simulink model "visual_sim"  (R2020a)
settings: Solver=ode3  StartTime=0.0  StopTime=Inf  RelTol=1e-3  EnableMultiTasking=on
undefined symbols (not defined in the file or in its folder): Rec, SDTV
libraries: dspsigops x6, simulink x3, visionstatistics x1, visionanalysis x1, visionconversions x1, embdlinuxlib x1
settings Model: FPTRunName=Active  ExtModeTrigDuration=2  Creator=ianli  LastModifiedBy=vyvo9
settings SolverCC: PositivePriorityOrder=on
settings DataIOCC: LimitDataPoints=on  SaveFormat=Array
settings OptimizationCC: ExpressionDepthLimit=2147483647  LifeSpan=Inf  MaxStackSize=64
settings DebuggingCC: UnderspecifiedInitializationDetection=Classic  MergeDetectMultiDrivingBlocksExec=none  FcnCallInpInsideContextMsg=warning  AllowSymbolicDim=off  StateNameClashWarn=warning  SFUnexpectedBacktrackingDiag=warning  SFNoUnconditionalDefaultTransitionDiag=warning  SFExecutionAtInitializationDiag=none  ArithmeticOperatorsInVariantConditions=warning
settings HardwareCC: ProdBitPerPointer=32  ProdBitPerSizeT=32  ProdBitPerPtrDiffT=32  ProdLargestAtomicInteger=Long  ProdLargestAtomicFloat=Double  ProdWordSize=32  ProdHWDeviceType=ARM Compatible->ARM Cortex  UseEmbeddedCoderFeatures=off
settings ModelReferenceCC: PropagateSignalLabelsOutOfModel=off
settings SFSimCC: SimUseLocalCustomCode=off  CustomCodeUndefinedFunction=UseInterfaceOnly
settings RTWCC: SystemTargetFile=ert.tlc  HardwareBoard=Raspberry Pi  TemplateMakefile=ert_default_tmf  GenerateReport=on  RTWVerbose=off  RTWUseLocalCustomCode=off  Toolchain=GNU GCC Raspberry Pi  BuildConfiguration=Faster Runs  LaunchReport=on
settings CodeAppCC: ForceParamTrailComments=on  OperatorAnnotations=on  StateflowObjectComments=on  MATLABSourceComments=on
settings ERTTargetCC: MultiwordLength=2048  ERTCustomFileBanners=off  SupportContinuousTime=on  SupportNonInlinedSFcns=on  RemoveResetFunc=off  SupportVariableSizeSignals=on  ModelStepFunctionPrototypeControlCompliant=off
settings ConfigComp: CovMetricSettings=dw  CovHtmlReporting=on  CovSaveCumulativeToWorkspaceVar=on  CovSaveSingleToWorkspaceVar=on  CovExternalEMLEnable=off  CovSFcnEnable=off

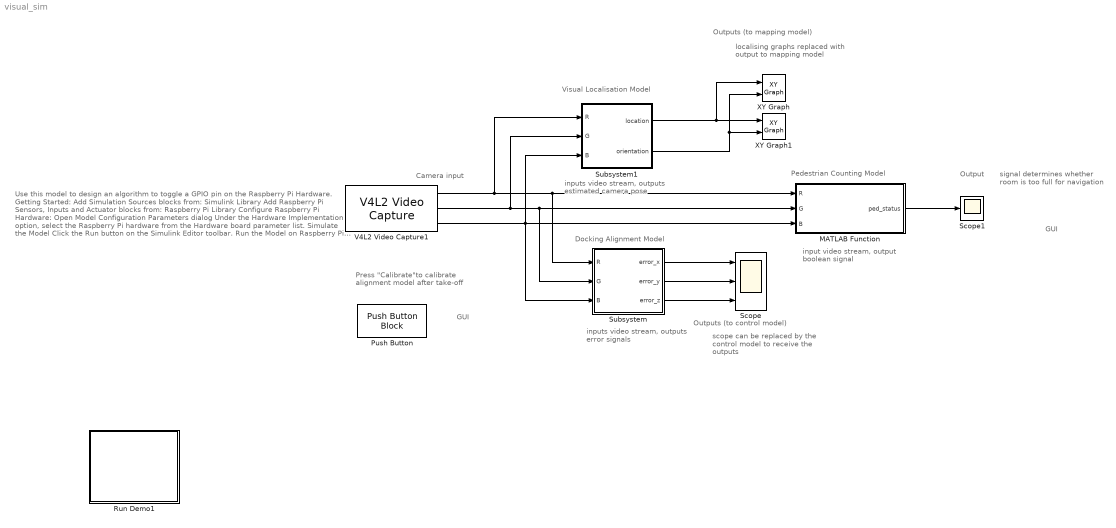
== system visual_sim ==
  note: Outputs (to control model)
  note: inputs video stream,
      | outputs error signals
  note: Camera input
  note: Docking Alignment Model
  note: Press "Calibrate"to calibrate alignment model after take-off
  note: scope can be replaced by the control model to receive the outputs
  note: GUI
  note: input video stream,
      | output boolean signal
  note: Use this model to design an algorithm to toggle a GPIO pin on the Raspberry Pi Hardware.
      |
      | Getting Started:
      |
      | Add Simulation Sources blocks from:
      | Simulink Library
      | Add Raspberry Pi Sensors, Inputs and Actuator blocks from:
      | Raspberry Pi Library
      |
      | Configure Raspberry Pi Hardware:
      |
      | Open Model Configuration Parameters dialog
      | Under the Hardware Implementation option, select the Raspberry Pi hardware from the Hardware board parameter list.
      |
      | Simulate the Model
      |
      | Click the Run button on the Simulink Editor toolbar.
      |
      | Run the Model on Raspberry Pi Hardware
      |
      | In the Hardware tab, click Build, Deploy & Start
      |
      | Other Things to Try:
      |
      | Create and run a model that repeatedly brightens and dims an LED. Hint: Use PWM block as an Raspberry Pi actuator.
  note: Visual Localisation Model
  note: inputs video stream,
      | outputs estimated camera pose
  note: Output
  note: signal determines whether room is too full for navigation
  note: Pedestrian Counting Model
  note: Outputs (to mapping model)
  note: localising graphs replaced with output to mapping model
  note: GUI
  MATLAB Function : MATLAB Function  TreatAsAtomicUnit=on
  Push Button : PushButtonBlock  ButtonText=Callibrate
  Run Demo1 : Subsystem  Description=Controls host-side RTDX processing.
      mask Display: pic=imread('raspberrypiBuildDeployAndStart.png');image(pic);
  Scope : Scope  NumInputPorts=3
  Scope1 : Scope
  Subsystem : Subsystem
  Subsystem1 : Subsystem
  V4L2 Video Capture1 : embdlinuxlib/V4L2 Video Capture  m_devName='/dev/video0'  roi=[0, 0, 640, 480]  imSizeSelection=640x480  imSize=[640, 480]  pixelFormat=RGB  pixelOrder=Planar  sampleTime=1/10  simOutput=Colorbars  blockPlatform=Raspberry Pi
      settings: SourceProductBaseCode=SC_BEAGLEBONE_BLUE,RASPPI
  XY Graph : simulink/Sinks/XY Graph  xmin=-1  xmax=1  ymin=-1  ymax=1  st=-1
  XY Graph1 : simulink/Sinks/XY Graph  xmin=-1  xmax=1  ymin=-1  ymax=1  st=-1
  wires:
  Subsystem/1(error_x) -> Scope/1
  Subsystem/2(error_y) -> Scope/2
  Subsystem/3(error_z) -> Scope/3
  V4L2 Video Capture1/2 -> Subsystem1/2(G), Subsystem/2(G), MATLAB Function/2(G)
  V4L2 Video Capture1/3 -> MATLAB Function/3(B), Subsystem/3(B), Subsystem1/3(B)
  V4L2 Video Capture1/1 -> Subsystem1/1(R), Subsystem/1(R), MATLAB Function/1(R)
  MATLAB Function/1(ped_status) -> Scope1/1
  Subsystem1/1(location) -> XY Graph1/1, XY Graph/1
  Subsystem1/2(orientation) -> XY Graph1/2, XY Graph/2

== system visual_sim/Run Demo1 ==

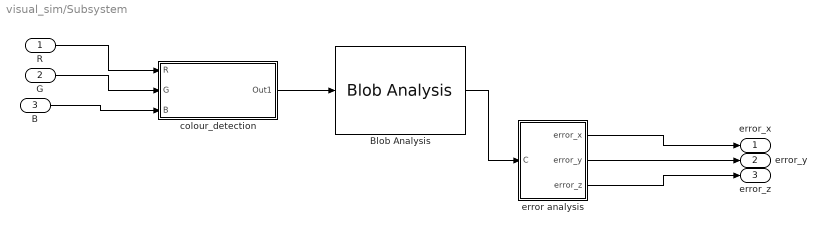
== system visual_sim/Subsystem ==
  R : Inport
  G : Inport  Port=2
  B : Inport  Port=3
  Blob Analysis : visionstatistics/Blob Analysis  Tag=vipblks_row_conv  area=off  centroid=on  bBox=off  majorAxis=off  minorAxis=off  angle=off  eccentricity=off  equivDiameterSq=off  extent=off  perimeter=off  outDT=double  conn=8  isLabel=off  maxBlobs=3  warnIfNumBlobsExceeded=on  isCount=off  useMinArea=off  minArea=0  useMaxArea=off  maxArea=intmax('uint32')  excludeBorderBlob=off  isOutVarDim=off  isFill=on  fillValues=-1  roundingMode=Floor  overflowMode=off  prodOutputMode=Binary point scaling  prodOutputWordLength=32  prodOutputFracLength=16  accumMode=Binary point scaling  accumWordLength=32  accumFracLength=0  outputMode=Binary point scaling  outputWordLength=32  outputFracLength=16  firstCoeffMode=Binary point scaling  firstCoeffWordLength=16  firstCoeffFracLength=14  secondCoeffMode=Binary point scaling  secondCoeffWordLength=32  secondCoeffFracLength=16
  colour_detection : Subsystem
  error analysis : Subsystem
  error_x : Outport
  error_y : Outport  Port=2
  error_z : Outport  Port=3
  wires:
  Blob Analysis/1 -> error analysis/1(C)
  colour_detection/1(Out1) -> Blob Analysis/1
  error analysis/1(error_x) -> error_x/1
  error analysis/2(error_y) -> error_y/1
  error analysis/3(error_z) -> error_z/1
  R/1 -> colour_detection/1(R)
  G/1 -> colour_detection/2(G)
  B/1 -> colour_detection/3(B)

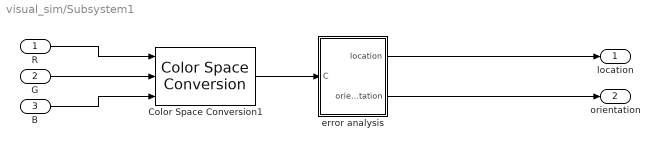
== system visual_sim/Subsystem1 ==
  R : Inport
  G : Inport  Port=2
  B : Inport  Port=3
  Color Space Conversion1 : visionconversions/Color Space  Conversion  conversion=Obsolete  conversionActive=R'G'B' to intensity  wp_str=D65  rec=Rec. 601 (SDTV)  sys=1125/60/2:1  imagePorts=Separate color signals
  error analysis : Subsystem
  location : Outport
  orientation : Outport  Port=2
  wires:
  error analysis/1(location) -> location/1
  error analysis/2(orientation) -> orientation/1
  R/1 -> Color Space Conversion1/1
  G/1 -> Color Space Conversion1/2
  B/1 -> Color Space Conversion1/3
  Color Space Conversion1/1 -> error analysis/1(C)

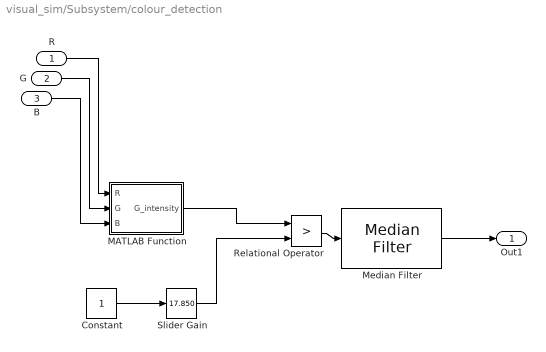
== system visual_sim/Subsystem/colour_detection ==
  R : Inport
  G : Inport  Port=2
  B : Inport  Port=3
  Constant : Constant
  MATLAB Function : MATLAB Function  TreatAsAtomicUnit=on
  Median Filter : visionanalysis/Median Filter  nghbood=[3 3]  outSize=Same as input port I  padType=Constant  padSrc=Specify via dialog  padVal=0  roundingMode=Floor  overflowMode=off
      settings: SourceProductBaseCode=VP
  Relational Operator : RelationalOperator  Operator=>  OutDataTypeStr=boolean  RndMeth=Simplest
  Slider Gain : simulink/Math Operations/Slider Gain  gain=17.850  low=0  high=255
  Out1 : Outport
  wires:
  Slider Gain/1 -> Relational Operator/2
  Constant/1 -> Slider Gain/1
  MATLAB Function/1(G_intensity) -> Relational Operator/1
  G/1 -> MATLAB Function/2(G)
  B/1 -> MATLAB Function/3(B)
  Median Filter/1 -> Out1/1
  R/1 -> MATLAB Function/1(R)
  Relational Operator/1 -> Median Filter/1

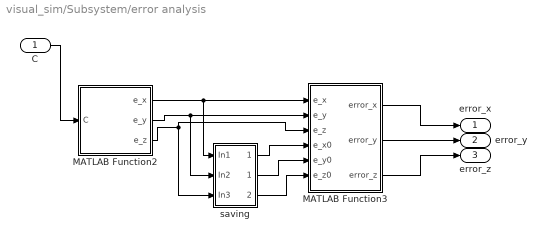
== system visual_sim/Subsystem/error analysis ==
  C : Inport
  MATLAB Function2 : MATLAB Function  TreatAsAtomicUnit=on
  MATLAB Function3 : MATLAB Function  TreatAsAtomicUnit=on
  saving : Subsystem
  error_x : Outport
  error_y : Outport  Port=2
  error_z : Outport  Port=3
  wires:
  MATLAB Function2/2(e_y) -> MATLAB Function3/2(e_y), saving/2(In2)
  MATLAB Function2/1(e_x) -> saving/1(In1), MATLAB Function3/1(e_x)
  saving/3(" 2") -> MATLAB Function3/6(e_z0)
  saving/2(" 1") -> MATLAB Function3/5(e_y0)
  MATLAB Function2/3(e_z) -> MATLAB Function3/3(e_z), saving/3(In3)
  saving/1(" ") -> MATLAB Function3/4(e_x0)
  MATLAB Function3/1(error_x) -> error_x/1
  MATLAB Function3/3(error_z) -> error_z/1
  MATLAB Function3/2(error_y) -> error_y/1
  C/1 -> MATLAB Function2/1(C)

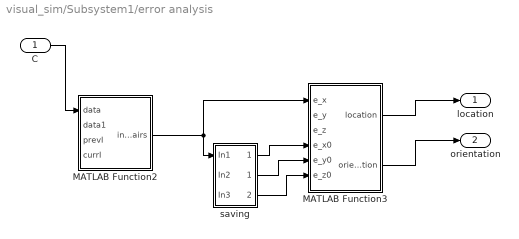
== system visual_sim/Subsystem1/error analysis ==
  C : Inport
  MATLAB Function2 : MATLAB Function  TreatAsAtomicUnit=on
  MATLAB Function3 : MATLAB Function  TreatAsAtomicUnit=on
  saving : Subsystem
  location : Outport
  orientation : Outport  Port=2
  wires:
  ? -> MATLAB Function3/2(e_y), saving/2(In2)
  MATLAB Function2/1(indexPairs) -> MATLAB Function3/1(e_x), saving/1(In1)
  saving/3(" 2") -> MATLAB Function3/6(e_z0)
  saving/2(" 1") -> MATLAB Function3/5(e_y0)
  ? -> MATLAB Function3/3(e_z), saving/3(In3)
  saving/1(" ") -> MATLAB Function3/4(e_x0)
  MATLAB Function3/1(location) -> location/1
  MATLAB Function3/2(orientation) -> orientation/1
  C/1 -> MATLAB Function2/1(data)

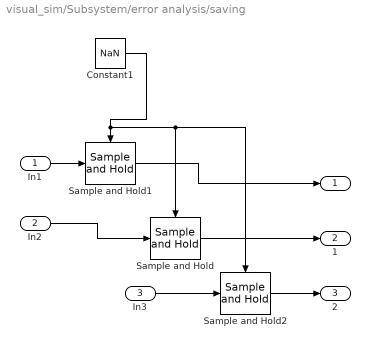
== system visual_sim/Subsystem/error analysis/saving ==
  In1 : Inport
  In2 : Inport  Port=2
  In3 : Inport  Port=3
  Constant1 : Constant  Value=NaN
  Sample and Hold : dspsigops/Sample and Hold  trig=Rising edge  initCond=0  latchinput=off
  Sample and Hold1 : dspsigops/Sample and Hold  trig=Rising edge  initCond=0  latchinput=off
  Sample and Hold2 : dspsigops/Sample and Hold  trig=Rising edge  initCond=0  latchinput=off
  " " : Outport
  " 1" : Outport  Port=2
  " 2" : Outport  Port=3
  wires:
  Sample and Hold1/1 -> " "/1
  In1/1 -> Sample and Hold1/1
  In2/1 -> Sample and Hold/1
  Sample and Hold/1 -> " 1"/1
  Sample and Hold2/1 -> " 2"/1
  In3/1 -> Sample and Hold2/1
  Constant1/1 -> Sample and Hold2/Trigger, Sample and Hold/Trigger, Sample and Hold1/Trigger

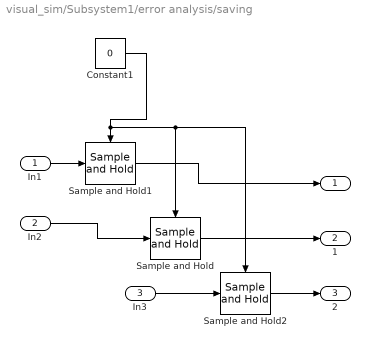
== system visual_sim/Subsystem1/error analysis/saving ==
  In1 : Inport
  In2 : Inport  Port=2
  In3 : Inport  Port=3
  Constant1 : Constant  Value=0
  Sample and Hold : dspsigops/Sample and Hold  trig=Rising edge  initCond=0  latchinput=off
  Sample and Hold1 : dspsigops/Sample and Hold  trig=Rising edge  initCond=0  latchinput=off
  Sample and Hold2 : dspsigops/Sample and Hold  trig=Rising edge  initCond=0  latchinput=off
  " " : Outport
  " 1" : Outport  Port=2
  " 2" : Outport  Port=3
  wires:
  Sample and Hold1/1 -> " "/1
  In1/1 -> Sample and Hold1/1
  In2/1 -> Sample and Hold/1
  Sample and Hold/1 -> " 1"/1
  Sample and Hold2/1 -> " 2"/1
  In3/1 -> Sample and Hold2/1
  Constant1/1 -> Sample and Hold2/Trigger, Sample and Hold/Trigger, Sample and Hold1/Trigger

== matlab function visual_sim/Subsystem/colour_detection/MATLAB Function ==
  data: R input; G_intensity output; G input; B input
function G_intensity  = fcn(R,G,B)

G_intensity = G - R./2 - B./2;

== matlab function visual_sim/Subsystem/error analysis/MATLAB Function2 ==
  data: C input; e_x output; e_y output; e_z output
function [e_x, e_y, e_z] = distances(C) % note everything is in pixels

% input C gives a 3-by-2 matrix in in the form [x1 y1 ; x2 y2 ; x3 y3] of
% the coordinates of the centroids
% (possible input that can be obtained from blob analysis is also blob area
% which can be used to identify the different blobs)
if length(C)==3
    C_sorted = sortrows(C); % sort so rows 1-3 correspond to blobs from L-R
    % NB blob 1,3 are the back markers, blob 3 is the front marker
    e_x = (C_sorted(3,1)+C_sorted(2,1))/2-C_sorted(2,1); %+ve error - too far right
    e_z = (C_sorted(3,2)+C_sorted(2,2))/2-C_sorted(2,2); %+ve error - too high
    e_y = (C_sorted(3,1)-C_sorted(1,1)); % relative distance between poles in pixels
end

== matlab function visual_sim/Subsystem/error analysis/MATLAB Function3 ==
  data: e_x input; e_y input; error_x output; error_y output; e_z input; e_x0 input; e_y0 input; e_z0 input; error_z output
function [error_x,error_y,error_z] = fcn(e_x,e_y,e_z,e_x0,e_y0,e_z0)

error_x = e_x-e_x0;
error_z = e_z-e_z0;
error_y = e_y-e_y0;

== matlab function visual_sim/MATLAB Function ==
  data: R input; ped_status output; G input; B input
function ped_status = PedestrianTracking(R, G, B)
[obj, tracks, full, FrameWithTracker] = PedestrianTracker();
objs = obj;
trackss = tracks;
ped_status = [full, FrameWithTracker];

== matlab function visual_sim/Subsystem1/error analysis/MATLAB Function2 ==
  data: data input; indexPairs output; data1 input; prevI input; currI input
function indexPairs  = fcn(data, data1, prevI, currI)

prevPoints = detectSURFFeatures(prevI, 'MetricThreshold', data);
prevPoints = selectUniform(prevPoints, data1, size(prevI));
prevFeatures = extractFeatures(prevI, prevPoints, 'Upright', true);

currPoints = detectSURFFeatures(currI, 'MetricThreshold', data);
currPoints = selectUniform(currPoints, data1, size(currI));
currFeatures = extractFeatures(currI, currPoints, 'Upright', true);

indexPairs = matchFeatures(prevFeatures, currFeatures, 'Unique', true);

matchedPoints1 = prevPoints(indexPairs(:,1));
matchedPoints2 = currPoints(indexPairs(:,2));

focalLength = [(3.6/0.0014) (3.6/0.0014)];
principalPoint = [320/2 240/2];  
imageSize      = [240 320];
intrinsics = cameraIntrinsics(focalLength, principalPoint, imageSize);

if ~isnumeric(matchedPoints1)
    matchedPoints1 = matchedPoints1.Location;
end

if ~isnumeric(matchedPoints2)
    matchedPoints2 = matchedPoints2.Location;
end

for i = 1:100
    % Estimate the essential matrix.    
    [E, inlierIdx] = estimateEssentialMatrix(matchedPoints1, matchedPoints2,...
        intrinsics);

    % Make sure we get enough inliers
    if sum(inlierIdx) / numel(inlierIdx) < .3
        continue;
    end
    
    % Get the epipolar inliers.
    inlierPoints1 = matchedPoints1(inlierIdx, :);
    inlierPoints2 = matchedPoints2(inlierIdx, :);    
    
    % Compute the camera pose from the fundamental matrix. Use half of the
    % points to reduce computation.
    [orientation, location, validPointFraction] = ...
        relativeCameraPose(E, intrinsics, inlierPoints1(1:2:end, :),...
        inlierPoints2(1:2:end, :));

    % validPointFraction is the fraction of inlier points that project in
    % front of both cameras. If the this fraction is too small, then the
    % fundamental matrix is likely to be incorrect.
    if validPointFraction > .8
       return;
    end
end

indexPairs = indexPairs(inlierIdx, :);

== matlab function visual_sim/Subsystem1/error analysis/MATLAB Function3 ==
  data: e_x input; e_y input; location output; orientation output; e_z input; e_x0 input; e_y0 input; e_z0 input
function [location, orientation] = fcn(e_x,e_y,e_z,e_x0,e_y0,e_z0)

location = e_x-e_x0;
orientation = e_z-e_z0;
